simulink model "LineariLQRmimo"  (R2021b)
settings: Solver=FixedStepDiscrete  StartTime=0.0  StopTime=10.0  FixedStep=0.001  MaxStep=0.001  RelTol=1e-3
undefined symbols (not defined in the file): A, B, Q, Qf, R
settings Model: Creator=USUARIO  LastModifiedBy=USUARIO

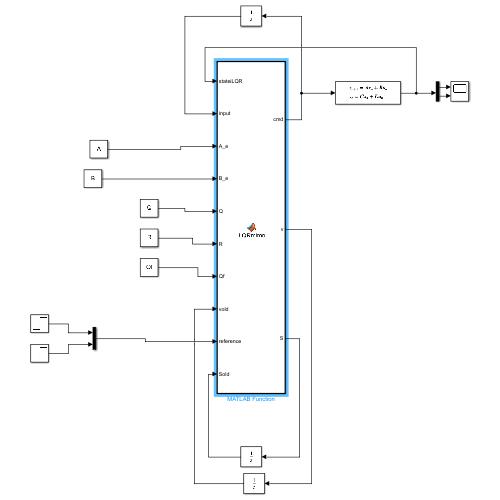
[thumbnail: Simulink's stored preview of the top-level diagram]
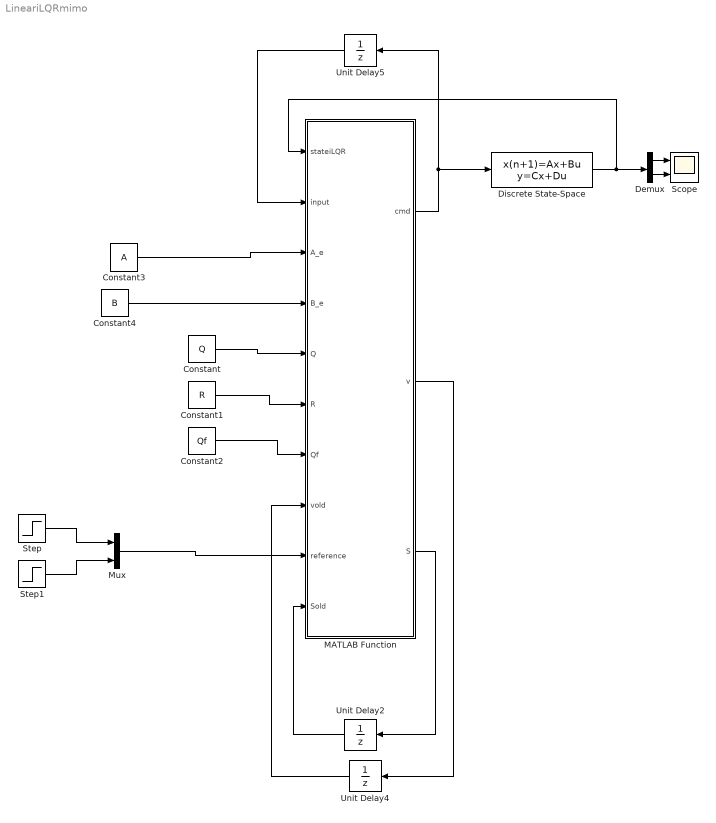
== system LineariLQRmimo ==
  Constant : Constant  Value=Q
  Constant1 : Constant  Value=R
  Constant2 : Constant  Value=Qf
  Constant3 : Constant  Value=A
  Constant4 : Constant  Value=B
  Demux : Demux  Outputs=2
  Discrete State-Space : DiscreteStateSpace  A=A  B=B  C=eye(2)  D=zeros(2)  SampleTime=-1
  MATLAB Function : MATLAB Function  TreatAsAtomicUnit=on
  Mux : Mux  Inputs=2
  Scope : Scope  NumInputPorts=2
  Step : Step  SampleTime=0
  Step1 : Step  SampleTime=0
  Unit Delay2 : UnitDelay  InitialCondition=Qf  SampleTime=-1  HasFrameUpgradeWarning=on
  Unit Delay4 : UnitDelay  InitialCondition=zeros(2,1)  SampleTime=-1  HasFrameUpgradeWarning=on
  Unit Delay5 : UnitDelay  InitialCondition=zeros(2,1)  SampleTime=-1  HasFrameUpgradeWarning=on
  wires:
  MATLAB Function/3(S) -> Unit Delay2/1
  Unit Delay2/1 -> MATLAB Function/10(Sold)
  MATLAB Function/2(v) -> Unit Delay4/1
  Unit Delay4/1 -> MATLAB Function/8(vold)
  Constant2/1 -> MATLAB Function/7(Qf)
  Constant1/1 -> MATLAB Function/6(R)
  Constant/1 -> MATLAB Function/5(Q)
  MATLAB Function/1(cmd) -> Unit Delay5/1, Discrete State-Space/1
  Discrete State-Space/1 -> MATLAB Function/1(stateiLQR), Demux/1
  Unit Delay5/1 -> MATLAB Function/2(input)
  Step/1 -> Mux/1
  Step1/1 -> Mux/2
  Mux/1 -> MATLAB Function/9(reference)
  Constant4/1 -> MATLAB Function/4(B_e)
  Constant3/1 -> MATLAB Function/3(A_e)
  Demux/1 -> Scope/1
  Demux/2 -> Scope/2

== matlab function LineariLQRmimo/MATLAB Function ==
  data: stateiLQR input; input input; A_e input; B_e input; cmd output; Q input; R input; Qf input; vold input; reference input; Sold input; v output; S output
function [cmd, v, S] = iLQRmimo(stateiLQR,input,A_e,B_e, Q, R, Qf, vold, reference, Sold)
% toll = 3*10^-5;

A = A_e;
B = B_e;
state = stateiLQR';
J = state*Qf*state'+state*Q*state'+input'*R*input;


% if abs(Jold-J)/Jold > toll
K  = (B'*Sold*B+R)\B'*Sold*A;
Kv = (B'*Sold*B+R)\B';
Ku = (B'*Sold*B+R)\R;
S  = A'*Sold*(A-B*K)+Q;
deltax = -reference; % Changed the sign on this one because
% otherwise, the state is mirrored to the reference
v  = (A-B*K)'*vold+Q*deltax-K'*R*input;
deltau = -K*state'-Kv*v-Ku*input;
cmd  = input + deltau;
